simulink model "Simulacion_control_pos_or_PD_2"  (R2024b)
settings: Solver=FixedStepAuto  StartTime=0.0  StopTime=15.0  FixedStep=1e-3  RelTol=1e-3
settings Model: Creator=Raul Robles  LastModifiedBy=Raul Robles

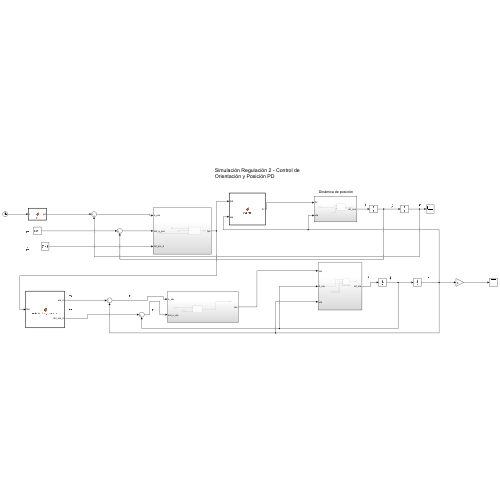
[thumbnail: Simulink's stored preview of the top-level diagram]
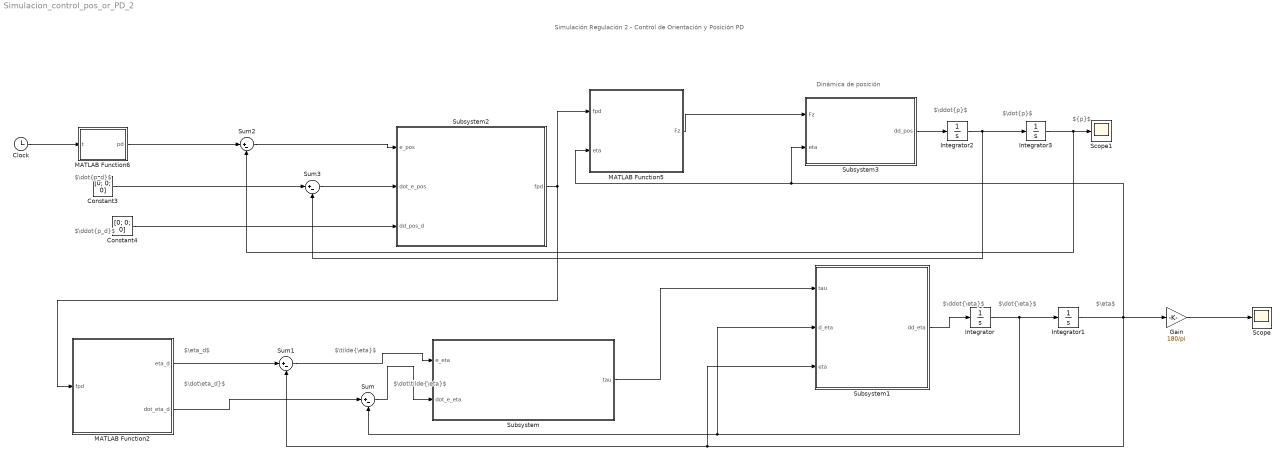
== system Simulacion_control_pos_or_PD_2 ==
  note: Simulación Regulación 2 - Control de Orientación y Posición PD
  note: $\eta$
  note: ${p}$
  note: $\ddot{p_d}$
  note: $\eta_d$
  note: $\dot{p}$
  note: $\tilde{\eta}$
  note: $\dot{p_d}$
  note: $\dot\eta_d}$
  note: $\dot\tilde{\eta}$
  note: $\dot{\eta}$
  note: Dinámica de posición
  note: $\ddot{\eta}$
  note: $\ddot{p}$
  Clock : Clock
      settings: Decimation=15
  Constant3 : Constant  Value=[0; 0; 0]
  Constant4 : Constant  Value=[0; 0; 0]
  Gain : Gain  Gain=180/pi
  Integrator{,1..3} (4 alike) : Integrator  InitialCondition=[0; 0; 0]
  MATLAB Function2 : MATLAB Function  TreatAsAtomicUnit=on
  MATLAB Function5 : MATLAB Function  TreatAsAtomicUnit=on
  MATLAB Function6 : MATLAB Function  TreatAsAtomicUnit=on
  Scope : Scope
  Scope1 : Scope
  Subsystem : Subsystem
  Subsystem1 : Subsystem
  Subsystem2 : Subsystem
  Subsystem3 : Subsystem
  Sum{,1..3} (4 alike) : Sum  Inputs=|+-
  wires:
  MATLAB Function2/1(eta_d) -> Sum1/1
  MATLAB Function2/2(dot_eta_d) -> Sum/1
  Integrator3/1 -> Sum2/2, Scope1/1
  Integrator1/1 -> Subsystem3/2(eta), MATLAB Function5/2(eta), Gain/1, Subsystem1/3(eta), Sum1/2
  Gain/1 -> Scope/1
  Integrator/1 -> Subsystem1/2(d_eta), Sum/2, Integrator1/1
  Integrator2/1 -> Integrator3/1, Sum3/2
  Constant3/1 -> Sum3/1
  Clock/1 -> MATLAB Function6/1(t)
  MATLAB Function6/1(pd) -> Sum2/1
  Sum1/1 -> Subsystem/1(e_eta)
  Sum/1 -> Subsystem/2(dot_e_eta)
  Subsystem/1(tau) -> Subsystem1/1(tau)
  Subsystem1/1(dd_eta) -> Integrator/1
  Subsystem2/1(fpd) -> MATLAB Function2/1(fpd), MATLAB Function5/1(fpd)
  Sum2/1 -> Subsystem2/1(e_pos)
  Sum3/1 -> Subsystem2/2(dot_e_pos)
  Constant4/1 -> Subsystem2/3(dd_pos_d)
  MATLAB Function5/1(Fz) -> Subsystem3/1(Fz)
  Subsystem3/1(dd_pos) -> Integrator2/1

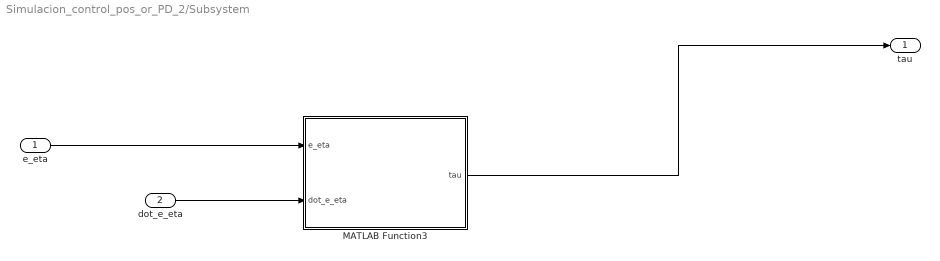
== system Simulacion_control_pos_or_PD_2/Subsystem ==
  e_eta : Inport
  dot_e_eta : Inport  Port=2
  MATLAB Function3 : MATLAB Function  TreatAsAtomicUnit=on
  tau : Outport
  wires:
  MATLAB Function3/1(tau) -> tau/1
  dot_e_eta/1 -> MATLAB Function3/2(dot_e_eta)
  e_eta/1 -> MATLAB Function3/1(e_eta)

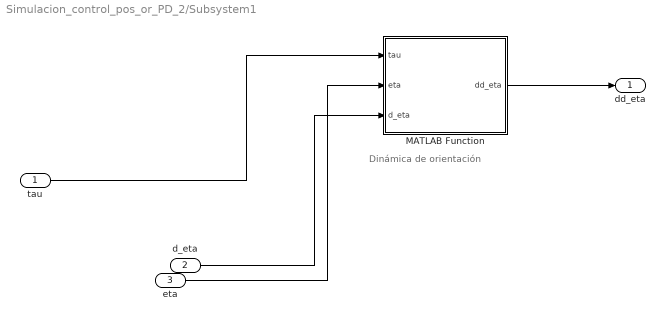
== system Simulacion_control_pos_or_PD_2/Subsystem1 ==
  note: Dinámica de orientación
  tau : Inport
  d_eta : Inport  Port=2
  eta : Inport  Port=3
  MATLAB Function : MATLAB Function  TreatAsAtomicUnit=on
  dd_eta : Outport
  wires:
  eta/1 -> MATLAB Function/2(eta)
  d_eta/1 -> MATLAB Function/3(d_eta)
  MATLAB Function/1(dd_eta) -> dd_eta/1
  tau/1 -> MATLAB Function/1(tau)

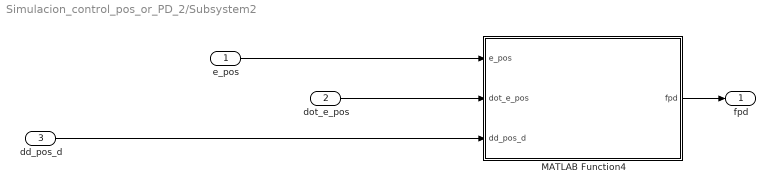
== system Simulacion_control_pos_or_PD_2/Subsystem2 ==
  e_pos : Inport
  dot_e_pos : Inport  Port=2
  dd_pos_d : Inport  Port=3
  MATLAB Function4 : MATLAB Function  TreatAsAtomicUnit=on
  fpd : Outport
  wires:
  dot_e_pos/1 -> MATLAB Function4/2(dot_e_pos)
  dd_pos_d/1 -> MATLAB Function4/3(dd_pos_d)
  e_pos/1 -> MATLAB Function4/1(e_pos)
  MATLAB Function4/1(fpd) -> fpd/1

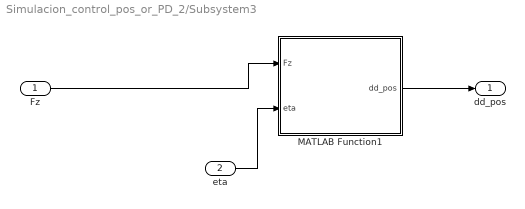
== system Simulacion_control_pos_or_PD_2/Subsystem3 ==
  Fz : Inport
  eta : Inport  Port=2
  MATLAB Function1 : MATLAB Function  TreatAsAtomicUnit=on
  dd_pos : Outport
  wires:
  Fz/1 -> MATLAB Function1/1(Fz)
  eta/1 -> MATLAB Function1/2(eta)
  MATLAB Function1/1(dd_pos) -> dd_pos/1

== matlab function Simulacion_control_pos_or_PD_2/Subsystem3/MATLAB Function1 ==
  data: Fz input; dd_pos output; eta input
function dd_pos = position_dynamics(Fz, eta)
    
%%% Masa del quad
m = 0.706; %%%[kg]

%%% Vector de gravedad
g = 9.81;
gz = [0; 0; g];

%%% Matriz de rotacion

R_11 = cos(eta(2))*cos(eta(3));
R_12 = sin(eta(1))*sin(eta(2))*cos(eta(3)) - cos(eta(1))*sin(eta(3));
R_13 = cos(eta(1))*sin(eta(2))*cos(eta(3)) + sin(eta(1))*sin(eta(3));
R_21 = cos(eta(2))*sin(eta(3));
R_22 = sin(eta(1))*sin(eta(2))*sin(eta(3)) + cos(eta(1))*cos(eta(3));
R_23 = cos(eta(1))*sin(eta(2))*sin(eta(3)) - sin(eta(1))*cos(eta(3));
R_31 = -sin(eta(2));
R_32 = sin(eta(1))*cos(eta(2));
R_33 = cos(eta(1))*cos(eta(2));

R = [R_11 R_12 R_13; R_21 R_22 R_23; R_31 R_32 R_33];

%%%% Vector r3

r3 = R*[0; 0; 1];

%%% Vector fp (fuerza en el marco de referencia inercial)

fp = r3*Fz;
% Dinámica de la posición
    dd_pos = (1/m)*fp - gz;
end

== matlab function Simulacion_control_pos_or_PD_2/Subsystem1/MATLAB Function ==
  data: tau input; dd_eta output; eta input; d_eta input
function dd_eta = orientation_dynamics(tau, eta, d_eta)
    
    % Matriz de inercia (momento de inercia)
    Ixx = 0.00273;
    Iyy = 0.00273;
    Izz = 0.00541;
    I = diag([Ixx, Iyy, Izz]);

    % Matriz de transformación PHI
    PHI_11 = 1;
    PHI_12 = sin(eta(1))*tan(eta(2));
    PHI_13 = cos(eta(1))*tan(eta(2));
    PHI_21 = 0;
    PHI_22 = cos(eta(1));
    PHI_23 = -sin(eta(1));
    PHI_31 = 0;
    PHI_32 = sin(eta(1))/cos(eta(2));
    PHI_33 = cos(eta(1))/cos(eta(2));

    PHI = [
        PHI_11, PHI_12, PHI_13;
        PHI_21, PHI_22, PHI_23;
        PHI_31, PHI_32, PHI_33
    ];
    
    % Derivada de la matriz PHI
    PHI_D_11 = 0;
    PHI_D_12 = d_eta(1)*cos(eta(1))*tan(eta(2)) + d_eta(2)*(sin(eta(1))/(cos(eta(2))^2));
    PHI_D_13 = d_eta(2)*(cos(eta(1))/(cos(eta(2))^2)) - d_eta(1)*sin(eta(1))*tan(eta(2));
    PHI_D_21 = 0;
    PHI_D_22 = -d_eta(1)*sin(eta(1));
    PHI_D_23 = -d_eta(1)*cos(eta(1));
    PHI_D_31 = 0;
    PHI_D_32 = (cos(eta(1))*cos(eta(2))*d_eta(1) + sin(eta(1))*sin(eta(2))*d_eta(2))/(cos(eta(2))^2);
    PHI_D_33 = (cos(eta(1))*sin(eta(2))*d_eta(2) - sin(eta(1))*cos(eta(2))*d_eta(1))/(cos(eta(2))^2);
    
    PHI_D = [
        PHI_D_11, PHI_D_12, PHI_D_13;
        PHI_D_21, PHI_D_22, PHI_D_23;
        PHI_D_31, PHI_D_32, PHI_D_33
    ];
    
   
    PHI_inv = inv(PHI); %%Inversa de la matriz PHI
    M = (PHI_inv') * I * PHI_inv; %%% Matriz M
    M_1 = inv(M); %%Inversa de la matriz M
    
    % Matriz S
    S = [0 -1 1; 1 0 -1; -1 1 0];
    
    % Matriz Coriolis
    C = (PHI_inv') * (S * (I * (PHI_inv)) - I * (PHI_inv) * PHI_D) * PHI_inv;
    
    fn = (PHI_inv') * tau; 

    % Cálculo de la aceleración angular
    dd_eta = (M_1) * (-C * d_eta + fn);
end

== matlab function Simulacion_control_pos_or_PD_2/MATLAB Function2 ==
  data: fpd input; eta_d output; dot_eta_d output
function [eta_d,dot_eta_d] = orientacion_deseada(fpd)

%%% Orientaciones deseadas y sus derivadas
psi_d = 0; %% Angulo psi deseado
dot_psi_d = 0; %% Derivada del angulo psi deseado

w = (1/fpd(3))*(fpd(2)*sin(psi_d) + fpd(1)*cos(psi_d));
theta_d = atan(w); %% Angulo theta deseado
dw = (1/fpd(3))*(fpd(2)*dot_psi_d*cos(psi_d) - fpd(1)*dot_psi_d*sin(psi_d)); 
dot_theta_d = (1/(1 + w*w))*dw; %% Derivada del angulo theta deseado

u = (cos(theta_d)/fpd(3))*(fpd(1)*sin(psi_d) - fpd(2)*cos(psi_d));
phi_d = atan(u); %%% Angulo phi deseado
du = (cos(psi_d)/fpd(3))*(fpd(1)*dot_psi_d*cos(psi_d) + fpd(2)*dot_psi_d*cos(psi_d)) - (dot_theta_d*sin(theta_d)/fpd(3))*(fpd(1)*sin(psi_d) - fpd(2)*cos(psi_d));
dot_phi_d = (1/(1 + u*u))*du;

eta_d = [phi_d; theta_d; psi_d];
dot_eta_d = [dot_phi_d; dot_theta_d; dot_psi_d];

== matlab function Simulacion_control_pos_or_PD_2/Subsystem/MATLAB Function3 ==
  data: e_eta input; tau output; dot_e_eta input
function tau = controller_orientation(e_eta,dot_e_eta)

v1 = [0.9 0.9 0.9];
v3 = [0.15 0.15 0.15];

%%% Ganancias de los controladores

Kp = diag(v1);
Kd = diag(v3);


tau = Kp*e_eta + Kd*dot_e_eta;

== matlab function Simulacion_control_pos_or_PD_2/Subsystem2/MATLAB Function4 ==
  data: e_pos input; dot_e_pos input; fpd output; dd_pos_d input
function fpd = controller_pos(e_pos, dot_e_pos,dd_pos_d)

%%% Masa del quad
m = 0.706;

%%% Gravedad
g = 9.81;

%%% Ganancias
Kpx = 3.9; %% Ganancia proporcional en x
Kpy = 3.9; %% Ganancia proporcional en y
Kpz = 11.7; %% Ganancia proporcional en z
Kdx = 1.95; %% Ganancia derivativa en x
Kdy = 1.95; %% Ganancia derivativa en y
Kdz = 3.325; %% Ganancia derivativa en z

fx_pd = m*dd_pos_d(1) + Kpx*e_pos(1) + Kdx*dot_e_pos(1);
fy_pd = m*dd_pos_d(2) + Kpy*e_pos(2) + Kdx*dot_e_pos(2);
fz_pd = m*dd_pos_d(3) + m*g + Kpy*e_pos(3) + Kdx*dot_e_pos(3);
fpd = [fx_pd; fy_pd; fz_pd];

== matlab function Simulacion_control_pos_or_PD_2/MATLAB Function5 ==
  data: fpd input; Fz output; eta input
function Fz = Fuerza(fpd,eta)

Fz = fpd(3)/(cos(eta(1))*cos(eta(2)));

== matlab function Simulacion_control_pos_or_PD_2/MATLAB Function6 ==
  data: t input; pd output
function pd = fn(t)
 
    if t >= 0 && t < 5
        pd = [0; 0; 0.8];
    elseif t >= 5 && t < 10
        pd = [0.3; 0.3; 0.8];
    elseif t >= 10 && t < 15
        pd = [-0.3; -0.3; 0.8];
    else
        pd = [0; 0; 0.8]; % O mantener la última posición
    end
end
